simulink model "Filtering_Test"  (R2024a)
settings: Solver=VariableStepAuto  StartTime=0.0  StopTime=10.0  RelTol=1e-3
undefined symbols (not defined in the file or in its folder): Amplitude_Wave_Lake, Factor_Wave_1, Factor_Wave_2, Frequency_Wave_Lake, Static_Gain_Waves
libraries: simulink x1
settings Model: Creator=gerar  LastModifiedBy=gerar

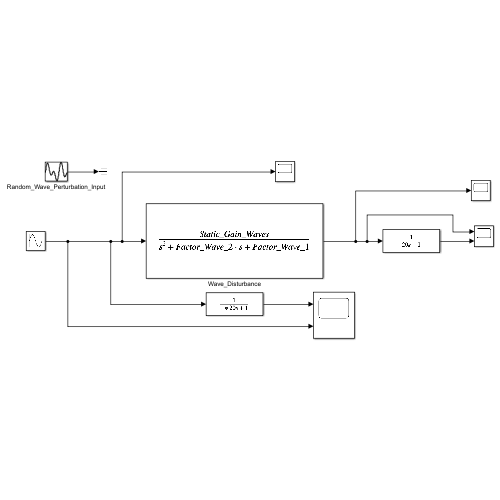
[thumbnail: Simulink's stored preview of the top-level diagram]
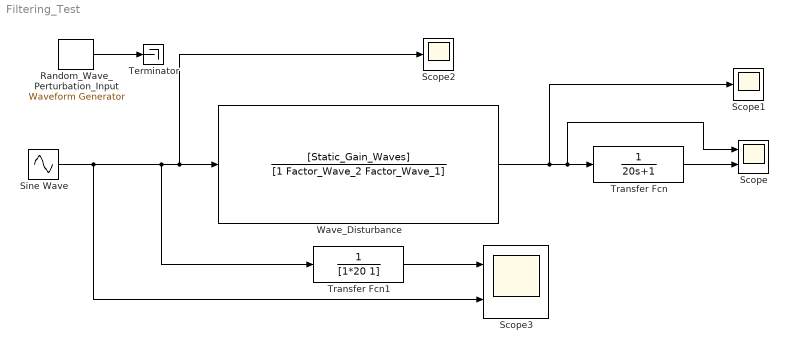
== system Filtering_Test ==
  Random_Wave_Perturbation_Input : simulink/Sources/Waveform Generator  OutMin=[]  OutMax=[]  OutDataTypeStr=double  SelectedSignal=1  Signals=sin(Amplitude_Wave_Lake, Frequency_Wave_Lake, 0)  BlockNames=MultiportSwitch_1a9f39972300416  SampleTime=0.1
  Scope : Scope  NumInputPorts=2
  Scope1 : Scope
  Scope2 : Scope
  Scope3 : Scope  NumInputPorts=2
  Sine Wave : Sin  Amplitude=15  Frequency=2*pi  SampleTime=0
  Terminator : Terminator
  Transfer Fcn : TransferFcn  Denominator=[20 1]
  Transfer Fcn1 : TransferFcn  Denominator=[1*20 1]
  Wave_Disturbance : TransferFcn  Numerator=[Static_Gain_Waves]  Denominator=[1 Factor_Wave_2 Factor_Wave_1]
  wires:
  Sine Wave/1 -> Scope3/2, Transfer Fcn1/1, Scope2/1, Wave_Disturbance/1
  Wave_Disturbance/1 -> Scope1/1, Scope/1, Transfer Fcn/1
  Random_Wave_Perturbation_Input/1 -> Terminator/1
  Transfer Fcn/1 -> Scope/2
  Transfer Fcn1/1 -> Scope3/1
